simulink model "dc_motor"  (R2017b)
settings: Solver=VariableStepAuto  StartTime=0.0  StopTime=1  MaxStep=1  RelTol=1e-6
libraries: simulink x2
settings Model: Creator=Administrator  LastModifiedBy=leiyang
settings CodeAppCC: StateflowObjectComments=on

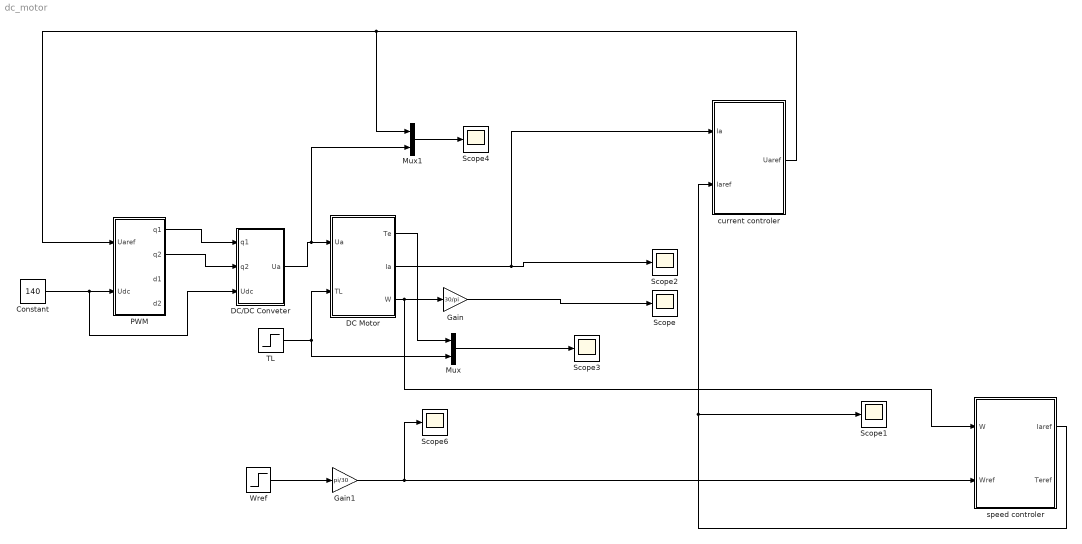
== system dc_motor ==
  Constant : Constant  Value=140
  DC Motor : Subsystem  mask{Ra=0.5, La=2.5e-3, J=1e-3, fr=5e-2, Ke=0.35, Kc=0.35}
      mask prompts: Ra "Ra(ohm)"; La "La(H)"; J "J(N.m.s^-1)"; fr "fr(N.m.s)"; Ke "Ke(V.s)"; Kc "Kc(N.m.A^1)"
  DC/DC Conveter : Subsystem
  Gain : Gain  Gain=30/pi
  Gain1 : Gain  Gain=pi/30
  Mux : Mux  Inputs=2
  Mux1 : Mux  Inputs=2
  PWM : Subsystem
  Scope{,1..4,6} (6 alike) : Scope
  TL : Step  Time=0.5  After=7  SampleTime=0
  Wref : Step  Time=0.1  After=2000  SampleTime=0
  current controler : Subsystem
  speed controler : Subsystem
  wires:
  DC Motor/3(W) -> speed controler/1(W), Gain/1
  PWM/1(q1) -> DC/DC Conveter/1(q1)
  PWM/2(q2) -> DC/DC Conveter/2(q2)
  DC/DC Conveter/1("Ua ") -> Mux1/2, DC Motor/1(Ua)
  TL/1 -> Mux/2, DC Motor/2("TL ")
  DC Motor/1(Te) -> Mux/1
  DC Motor/2(Ia) -> current controler/1(Ia), Scope2/1
  Gain/1 -> Scope/1
  Constant/1 -> DC/DC Conveter/3(Udc), PWM/2("Udc ")
  Mux/1 -> Scope3/1
  Mux1/1 -> Scope4/1
  Wref/1 -> Gain1/1
  Gain1/1 -> Scope6/1, speed controler/2(Wref)
  speed controler/1(Iaref) -> Scope1/1, current controler/2(Iaref)
  current controler/1(Uaref) -> Mux1/1, PWM/1("Uaref ")

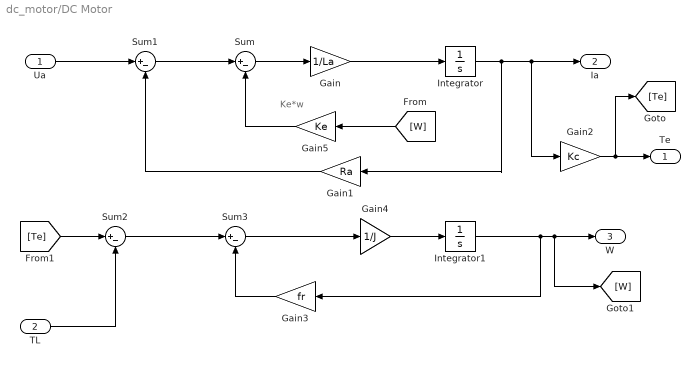
== system dc_motor/DC Motor ==
  note: Ke*w
  Ua : Inport
  "TL " : Inport  Port=2
  Gain : Gain  Gain=1/La
  Gain1 : Gain  Gain=Ra
  Gain2 : Gain  Gain=Kc
  Gain3 : Gain  Gain=fr
  Gain4 : Gain  Gain=1/J
  Gain5 : Gain  Gain=Ke
  Integrator : Integrator
  Integrator1 : Integrator
  Sum{,1..3} (4 alike) : Sum  Inputs=|+-
  Te : Outport
  Ia : Outport  Port=2
  W : Outport  Port=3
  wires:
  [W] -> Gain5/1
  Integrator1/1 -> Gain3/1, W/1, [W]
  Integrator/1 -> Gain1/1, Ia/1, Gain2/1
  Gain5/1 -> Sum/2
  Sum3/1 -> Gain4/1
  "TL "/1 -> Sum2/2
  Sum2/1 -> Sum3/1
  Gain/1 -> Integrator/1
  Sum/1 -> Gain/1
  [Te] -> Sum2/1
  Gain3/1 -> Sum3/2
  Gain4/1 -> Integrator1/1
  Ua/1 -> Sum1/1
  Gain1/1 -> Sum1/2
  Sum1/1 -> Sum/1
  Gain2/1 -> Te/1, [Te]

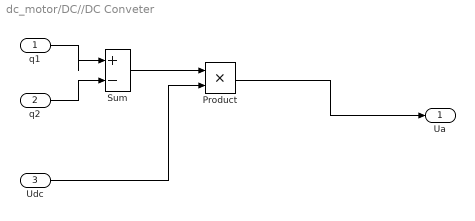
== system dc_motor/DC//DC Conveter ==
  q1 : Inport
  q2 : Inport  Port=2
  Udc : Inport  Port=3
  Product : Product
  Sum : Sum  Inputs=|+-
  "Ua " : Outport
  wires:
  q1/1 -> Sum/1
  q2/1 -> Sum/2
  Sum/1 -> Product/1
  Udc/1 -> Product/2
  Product/1 -> "Ua "/1

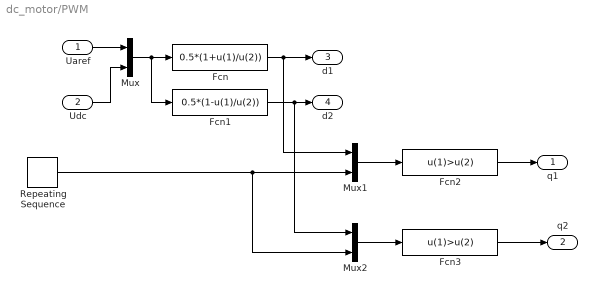
== system dc_motor/PWM ==
  "Uaref " : Inport
  "Udc " : Inport  Port=2
  Fcn : Fcn  Expr=0.5*(1+u(1)/u(2))
  Fcn1 : Fcn  Expr=0.5*(1-u(1)/u(2))
  Fcn2 : Fcn  Expr=u(1)>u(2)
  Fcn3 : Fcn  Expr=u(1)>u(2)
  Mux : Mux  Inputs=2
  Mux1 : Mux  Inputs=2
  Mux2 : Mux  Inputs=2
  Repeating Sequence : simulink/Sources/Repeating Sequence  rep_seq_t=[0 100e-6 200e-6]  rep_seq_y=[1 0 1]
  q1 : Outport
  q2 : Outport  Port=2
  d1 : Outport  Port=3
  d2 : Outport  Port=4
  wires:
  "Uaref "/1 -> Mux/1
  "Udc "/1 -> Mux/2
  Mux/1 -> Fcn1/1, Fcn/1
  Fcn/1 -> Mux1/1, d1/1
  Fcn1/1 -> Mux2/1, d2/1
  Repeating Sequence/1 -> Mux2/2, Mux1/2
  Mux1/1 -> Fcn2/1
  Mux2/1 -> Fcn3/1
  Fcn2/1 -> q1/1
  Fcn3/1 -> q2/1

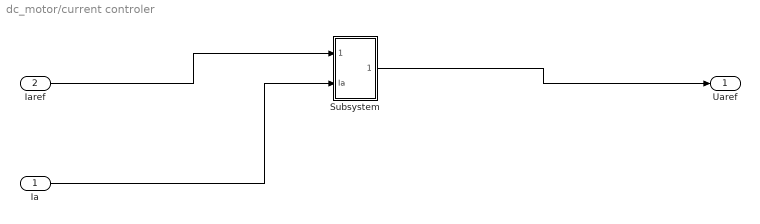
== system dc_motor/current controler ==
  Ia : Inport
  Iaref : Inport  Port=2
  Subsystem : Subsystem
  Uaref : Outport
  wires:
  Iaref/1 -> Subsystem/1(Iaref)
  Ia/1 -> Subsystem/2(Ia)
  Subsystem/1(Uaref) -> Uaref/1

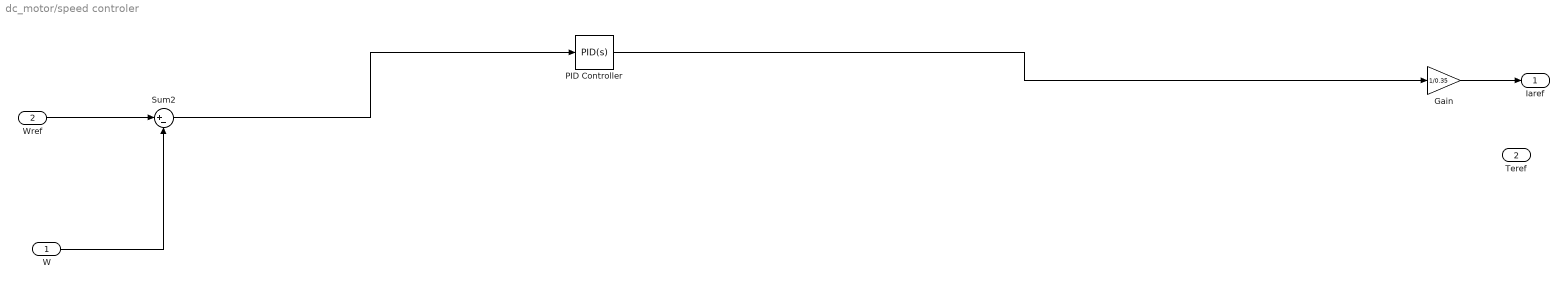
== system dc_motor/speed controler ==
  W : Inport
  Wref : Inport  Port=2
  Gain : Gain  Gain=1/0.35
  PID Controller : simulink/Continuous/PID Controller  Controller=PID  TimeDomain=Continuous-time  SampleTime=-1  IntegratorMethod=Forward Euler  FilterMethod=Forward Euler  Form=Parallel  UseFilter=on  ControllerParametersSource=internal  P=3  I=1.35  D=0  N=100  InitialConditionSource=internal  InitialConditionForIntegrator=0  InitialConditionForFilter=0  ExternalReset=none  LimitOutput=off  UpperSaturationLimit=inf  LowerSaturationLimit=-inf  LinearizeAsGain=on  AntiWindupMode=none  Kb=1  TrackingMode=off  Kt=1  PParamMin=[]  PParamMax=[]  IParamMin=[]  IParamMax=[]  DParamMin=[]  DParamMax=[]  NParamMin=[]  NParamMax=[]  KbParamMin=[]  KbParamMax=[]  KtParamMin=[]  KtParamMax=[]  POutMin=[]  POutMax=[]  IOutMin=[]  IOutMax=[]  DOutMin=[]  DOutMax=[]  NOutMin=[]  NOutMax=[]  KbOutMin=[]  KbOutMax=[]  KtOutMin=[]  KtOutMax=[]  IntegratorOutMin=[]  IntegratorOutMax=[]  FilterOutMin=[]  FilterOutMax=[]  SumOutMin=[]  SumOutMax=[]  SumI1OutMin=[]  SumI1OutMax=[]  SumI2OutMin=[]  SumI2OutMax=[]  SumI3OutMin=[]  SumI3OutMax=[]  SumDOutMin=[]  SumDOutMax=[]  SaturationOutMin=[]  SaturationOutMax=[]  IntegratorContinuousStateAttributes=''  IntegratorStateMustResolveToSignalObject=off  IntegratorRTWStateStorageClass=Auto  FilterContinuousStateAttributes=''  FilterStateMustResolveToSignalObject=off  FilterRTWStateStorageClass=Auto  DifferentiatorICPrevScaledInput=0  DifferentiatorOutMin=[]  DifferentiatorOutMax=[]  InitialConditionSetting=State (most efficient)  FilterDiffOutCoefMin=[]  FilterDiffOutCoefMax=[]  SumDenOutMin=[]  SumDenOutMax=[]  SumNumOutMin=[]  SumNumOutMax=[]  ReciprocalOutMin=[]  ReciprocalOutMax=[]  DivideOutMin=[]  DivideOutMax=[]  TunerSelectOption=Transfer Function Based (PID Tuner App)
  Sum2 : Sum  Inputs=|+-
  Iaref : Outport
  Teref : Outport  Port=2
  wires:
  Gain/1 -> Iaref/1
  W/1 -> Sum2/2
  Wref/1 -> Sum2/1
  Sum2/1 -> PID Controller/1
  PID Controller/1 -> Gain/1

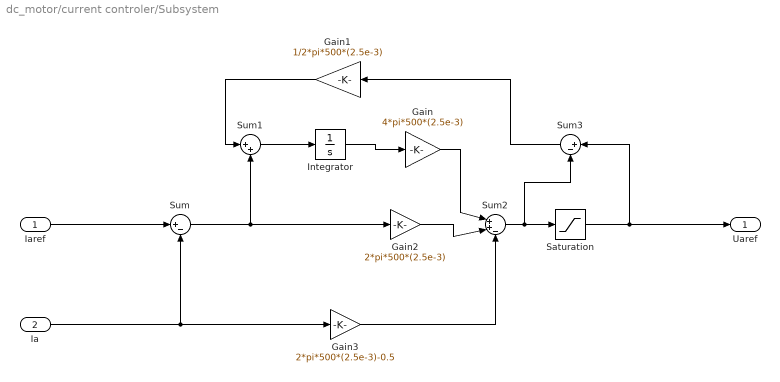
== system dc_motor/current controler/Subsystem ==
  Iaref : Inport
  Ia : Inport  Port=2
  Gain : Gain  Gain=4*pi*500*(2.5e-3)
  Gain1 : Gain  Gain=1/2*pi*500*(2.5e-3)
  Gain2 : Gain  Gain=2*pi*500*(2.5e-3)
  Gain3 : Gain  Gain=2*pi*500*(2.5e-3)-0.5
  Integrator : Integrator
  Saturation : Saturate  UpperLimit=140  LowerLimit=-140
  Sum : Sum  Inputs=|+-
  Sum1 : Sum  Inputs=|++
  Sum2 : Sum  Inputs=|++-
  Sum3 : Sum  Inputs=|+-
  Uaref : Outport
  wires:
  Gain/1 -> Sum2/1
  Gain2/1 -> Sum2/2
  Sum1/1 -> Integrator/1
  Gain3/1 -> Sum2/3
  Sum3/1 -> Gain1/1
  Ia/1 -> Gain3/1, Sum/2
  Sum/1 -> Gain2/1, Sum1/2
  Saturation/1 -> Uaref/1, Sum3/1
  Iaref/1 -> Sum/1
  Integrator/1 -> Gain/1
  Sum2/1 -> Sum3/2, Saturation/1
  Gain1/1 -> Sum1/1
